simulink model "lane_keeping_fpga_in_the_loop"  (R2025b)
settings: Solver=ode1  StartTime=0.0  StopTime=30.0  RelTol=1e-3
model workspace (MAT data in the model file):
  firstWarning = 1
  originalScenarioChecksum = '9B63FD3C04BCEB1F00254244C35DE55B'
undefined symbols (not defined in the file): gray, Sim3dSensor
libraries: instrumentseriallib x3, simulink_extras x2, visiongeotforms x1, sim3dcameralib x1, sim3dlib x1, sim3dautolib x1
(part 2 of 2)

== matlab function lane_keeping_fpga_in_the_loop/LANE KEEPING PROCESS/lane_mask_corsia ==
  data: binary_img input; lane_mask output
function lane_mask = Keep_First_White_Point(binary_img)
%#codegen
% Input : binary_img [H x W] uint8
% Output: lane_mask [H x W] uint8
%
% Scopo:
%   Estrarre le due linee di corsia anche se entrambe si trovano
%   nella stessa metà dell'immagine.
%
% Convenzioni:
%   r = riga immagine, cresce verso il basso
%   c = colonna immagine, cresce verso destra
%   centro corsia = media delle due linee oppure linea singola +/- mezza corsia

[H,W] = size(binary_img);

lane_mask = zeros(H,W,'uint8');

% =========================================================
% Memoria centro dinamico tra frame
% =========================================================
persistent center_mem initialized

if isempty(initialized)
    center_mem = int32(W/2);
    initialized = true;
end

% =========================================================
% Parametri
% =========================================================
pixels_per_meter_x = 30.0;    % [px/m]
lane_width_m       = 3.5;     % [m]

lane_width_px = int32(round(lane_width_m * pixels_per_meter_x));
half_lane_px  = int32(round(0.5 * double(lane_width_px)));

% Accetto linee entro questa distanza dal centro stimato
% Più grande di una corsia perché la macchina può essere disallineata.
search_gate_px = int32(round(2.2 * double(lane_width_px)));

% Tolleranza sulla larghezza corsia
width_tol_px = 0.45 * double(lane_width_px);

% Salto massimo ammesso tra una riga e la successiva
max_shift = int32(round(0.18 * double(W)));

% Aggiornamento lento del centro per evitare oscillazioni
alpha_center = 0.10;

% Numero massimo di blob candidati per riga
MAX_CAND = 20;

% Memoria intra-frame
prev_left  = int32(0);
prev_right = int32(0);

has_left  = false;
has_right = false;

center = center_mem;

% =========================================================
% Scansione dal basso verso l'alto
% =========================================================
for r = H:-1:1

    % Saturazione centro
    if center < 1
        center = int32(1);
    end
    if center > W
        center = int32(W);
    end

    % =====================================================
    % 1) Trova tutti i blob bianchi sulla riga r
    % =====================================================
    cand = zeros(1,MAX_CAND,'int32');
    cand_count = int32(0);

    in_blob = false;
    blob_start = int32(0);

    for c = 1:W

        is_white = binary_img(r,c) > 0;

        if is_white && ~in_blob
            in_blob = true;
            blob_start = int32(c);
        end

        if (~is_white || c == W) && in_blob

            if is_white && c == W
                blob_end = int32(c);
            else
                blob_end = int32(c - 1);
            end

            blob_center = int32(round(0.5 * ...
                (double(blob_start) + double(blob_end))));

            if cand_count < MAX_CAND
                cand_count = cand_count + 1;
                cand(cand_count) = blob_center;
            end

            in_blob = false;
        end
    end

    % Se non ho candidati, mantengo centro precedente
    if cand_count == 0
        continue;
    end

    % =====================================================
    % 2) Selezione delle due linee migliori
    % =====================================================
    best_left  = int32(0);
    best_right = int32(0);
    found_pair = false;

    best_pair_cost = 1.0e12;

    % -----------------------------------------------------
    % Caso A: cerco una coppia con distanza circa lane_width_px
    % -----------------------------------------------------
    for i = 1:cand_count
        ci = cand(i);

        % Scarto candidati troppo lontani dal centro dinamico
        if abs(ci - center) > search_gate_px
            continue;
        end

        for j = 1:cand_count
            if j <= i
                continue;
            end

            cj = cand(j);

            if abs(cj - center) > search_gate_px
                continue;
            end

            % Ordino: left < right
            if ci < cj
                c_left  = ci;
                c_right = cj;
            else
                c_left  = cj;
                c_right = ci;
            end

            width_px = c_right - c_left;

            % Deve essere circa una larghezza corsia
            width_error = abs(double(width_px) - double(lane_width_px));

            if width_error > width_tol_px
                continue;
            end

            pair_center = int32(round(0.5 * ...
                (double(c_left) + double(c_right))));

            % Costo geometrico
            cost_width  = width_error;
            cost_center = abs(double(pair_center - center));

            % Costo di continuità se ho memoria
            cost_cont = 0.0;

            if has_left
                if abs(c_left - prev_left) > max_shift
                    cost_cont = cost_cont + 1.0e6;
                else
                    cost_cont = cost_cont + abs(double(c_left - prev_left));
                end
            end

            if has_right
                if abs(c_right - prev_right) > max_shift
                    cost_cont = cost_cont + 1.0e6;
                else
                    cost_cont = cost_cont + abs(double(c_right - prev_right));
                end
            end

            total_cost = 4.0*cost_width + 1.0*cost_center + 2.0*cost_cont;

            if total_cost < best_pair_cost
                best_pair_cost = total_cost;
                best_left  = c_left;
                best_right = c_right;
                found_pair = true;
            end
        end
    end

    % =====================================================
    % 3) Se non trovo coppia, scelgo la singola linea migliore
    % =====================================================
    found_single = false;
    best_single = int32(0);
    best_single_cost = 1.0e12;

    if ~found_pair

        for i = 1:cand_count
            ci = cand(i);

            if abs(ci - center) > search_gate_px
                continue;
            end

            % Costo base: vicinanza al centro dinamico
            cost = abs(double(ci - center));

            % Se ho una linea precedente, privilegio la continuità
            if has_left && has_right
                dL = abs(ci - prev_left);
                dR = abs(ci - prev_right);
                cost = cost + 2.0 * double(min(dL,dR));
            elseif has_left
                cost = cost + 2.0 * double(abs(ci - prev_left));
            elseif has_right
                cost = cost + 2.0 * double(abs(ci - prev_right));
            end

            if cost < best_single_cost
                best_single_cost = cost;
                best_single = ci;
                found_single = true;
            end
        end
    end

    % =====================================================
    % 4) Scrittura output e aggiornamento centro
    % =====================================================
    center_new = center;

    if found_pair

        % Disegno entrambe le linee
        lane_mask(r,best_left)  = uint8(255);
        lane_mask(r,best_right) = uint8(255);

        prev_left  = best_left;
        prev_right = best_right;

        has_left  = true;
        has_right = true;

        center_new = int32(round(0.5 * ...
            (double(best_left) + double(best_right))));

    elseif found_single

        % Disegno la singola linea trovata
        lane_mask(r,best_single) = uint8(255);

        % Devo decidere se è linea sinistra o destra della corsia.
        % Ipotesi:
        %   se la linea è a sinistra del centro stimato, allora è left;
        %   se è a destra, allora è right.
        %
        % Nota: anche se entrambe le linee stanno nella stessa metà immagine,
        % questa scelta resta coerente rispetto al centro dinamico stimato.

        if best_single < center

            % Linea sinistra vista
            prev_left = best_single;
            has_left = true;

            center_new = best_single + half_lane_px;

        else

            % Linea destra vista
            prev_right = best_single;
            has_right = true;

            center_new = best_single - half_lane_px;

        end

    else

        center_new = center;

    end

    % =====================================================
    % 5) Filtro del centro dinamico
    % =====================================================
    center = int32(round((1.0 - alpha_center)*double(center) + ...
                         alpha_center*double(center_new)));

    if center < 1
        center = int32(1);
    end
    if center > W
        center = int32(W);
    end

end

% =========================================================
% Salvo memoria per frame successivo
% =========================================================
center_mem = center;

end

== matlab function lane_keeping_fpga_in_the_loop/LANE KEEPING PROCESS/rotazione corsia/fitting_lnes ==
  data: lane_img output; lane_mask input; validL output; aL output; bL output; cL output; validR output; aR output; bR output; cR output
function [lane_img, validL, aL, bL, cL, validR, aR, bR, cR] = Fit_Left_Right_Lanes(lane_mask)
%#codegen

[H,W] = size(lane_mask);
lane_img = lane_mask;

center_fixed = double(W)/2.0;

validL = false;
validR = false;

aL = 0.0;
bL = 0.0;
cL = 0.0;

aR = 0.0;
bR = 0.0;
cR = 0.0;

[validL1, validR1, aL1, bL1, cL1, aR1, bR1, cR1] = ...
    fit_lanes_internal(lane_mask, false, ...
                       0.0, 0.0, 0.0, ...
                       0.0, 0.0, 0.0, ...
                       center_fixed);

if ~(validL1 && validR1)

    validL = validL1;
    validR = validR1;

    aL = aL1;
    bL = bL1;
    cL = cL1;

    aR = aR1;
    bR = bR1;
    cR = cR1;

    return;
end

[validL2, validR2, aL2, bL2, cL2, aR2, bR2, cR2] = ...
    fit_lanes_internal(lane_mask, true, ...
                       aL1, bL1, cL1, ...
                       aR1, bR1, cR1, ...
                       center_fixed);

if validL2 && validR2

    validL = validL2;
    validR = validR2;

    aL = aL2;
    bL = bL2;
    cL = cL2;

    aR = aR2;
    bR = bR2;
    cR = cR2;

else

    validL = validL1;
    validR = validR1;

    aL = aL1;
    bL = bL1;
    cL = cL1;

    aR = aR1;
    bR = bR1;
    cR = cR1;

end

end


function [validL, validR, aL, bL, cL, aR, bR, cR] = ...
    fit_lanes_internal(lane_mask, use_corrected_center, ...
                       aLprev, bLprev, cLprev, ...
                       aRprev, bRprev, cRprev, ...
                       center_fixed)
%#codegen

persistent center_mem initialized

[H,W] = size(lane_mask);

if isempty(initialized)
    center_mem = center_fixed;
    initialized = true;
end

validL = false;
validR = false;

aL = 0.0;
bL = 0.0;
cL = 0.0;

aR = 0.0;
bR = 0.0;
cR = 0.0;

% =========================================================
% Parametri fisici
% =========================================================
pixels_per_meter_x = 30.0;
lane_width_m       = 3.5;

lane_width_px      = lane_width_m * pixels_per_meter_x;
half_lane_width_px = 0.5 * lane_width_px;

% Tolleranza per capire se distanza = 1 corsia o 2 corsie
width_tol_px = 0.35 * lane_width_px;

% Gate: accetto punti entro 1 corsia dal centro stimato
center_gate_px = lane_width_px;

% Media mobile centro
alpha_center = 0.20;

% =========================================================
% Accumulatori sinistra
% =========================================================
nL = 0.0;
SyL = 0.0;
Sy2L = 0.0;
Sy3L = 0.0;
Sy4L = 0.0;
SxL = 0.0;
SxyL = 0.0;
Sxy2L = 0.0;

% =========================================================
% Accumulatori destra
% =========================================================
nR = 0.0;
SyR = 0.0;
Sy2R = 0.0;
Sy3R = 0.0;
Sy4R = 0.0;
SxR = 0.0;
SxyR = 0.0;
Sxy2R = 0.0;

for r = 1:H

    y = double(r);

    if use_corrected_center

        xLprev = aLprev*y*y + bLprev*y + cLprev;
        xRprev = aRprev*y*y + bRprev*y + cRprev;

        measured_width = xRprev - xLprev;

        is_one_lane = abs(measured_width - lane_width_px) <= width_tol_px;
        is_two_lane = abs(measured_width - 2.0*lane_width_px) <= width_tol_px;

        if is_one_lane

            % Caso corretto: due linee della stessa corsia
            center_fit = 0.5*(xLprev + xRprev);

        elseif is_two_lane

            % Caso esterno: le due linee sono separate da circa 2 corsie
            dist_to_left  = abs(center_mem - xLprev);
            dist_to_right = abs(center_mem - xRprev);

            if dist_to_right < dist_to_left
                % linea più vicina è la destra:
                % centro corsia = mezzo lane width a sinistra della destra
                center_fit = xRprev - half_lane_width_px;
            else
                % linea più vicina è la sinistra:
                % centro corsia = mezzo lane width a destra della sinistra
                center_fit = xLprev + half_lane_width_px;
            end

        else

            % Caso incerto: mantengo memoria
            center_fit = center_mem;

        end

        % Media mobile
        center_mem = (1.0 - alpha_center)*center_mem + alpha_center*center_fit;

        center_dyn = center_mem;

        if center_dyn < 1.0
            center_dyn = 1.0;
        end

        if center_dyn > double(W)
            center_dyn = double(W);
        end

    else

        center_dyn = center_fixed;

    end

    for col = 1:W

        if lane_mask(r,col) > 0

            x = double(col);

            y2 = y*y;
            y3 = y2*y;
            y4 = y2*y2;

            assign_left = false;
            assign_right = false;

            if ~use_corrected_center

                if x < center_dyn
                    assign_left = true;
                else
                    assign_right = true;
                end

            else

                dist_from_center = abs(x - center_dyn);

                if dist_from_center <= center_gate_px

                    if x < center_dyn
                        assign_left = true;
                    else
                        assign_right = true;
                    end

                end
            end

            if assign_left

                nL = nL + 1.0;

                SyL   = SyL   + y;
                Sy2L  = Sy2L  + y2;
                Sy3L  = Sy3L  + y3;
                Sy4L  = Sy4L  + y4;

                SxL   = SxL   + x;
                SxyL  = SxyL  + x*y;
                Sxy2L = Sxy2L + x*y2;

            elseif assign_right

                nR = nR + 1.0;

                SyR   = SyR   + y;
                Sy2R  = Sy2R  + y2;
                Sy3R  = Sy3R  + y3;
                Sy4R  = SyR + y4;   % CORRETTO SOTTO
                Sy4R  = Sy4R - SyR + y4;

                SxR   = SxR   + x;
                SxyR  = SxyR  + x*y;
                Sxy2R = Sxy2R + x*y2;

            end
        end
    end
end

if nL >= 6.0

    [okL, aaL, bbL, ccL] = solve_parabola_ls( ...
        SyL, Sy2L, Sy3L, Sy4L, ...
        SxL, SxyL, Sxy2L, nL);

    if okL
        aL = aaL;
        bL = bbL;
        cL = ccL;
        validL = true;
    end
end

if nR >= 6.0

    [okR, aaR, bbR, ccR] = solve_parabola_ls( ...
        SyR, Sy2R, Sy3R, Sy4R, ...
        SxR, SxyR, Sxy2R, nR);

    if okR
        aR = aaR;
        bR = bbR;
        cR = ccR;
        validR = true;
    end
end

end


function [ok, a, b, c] = solve_parabola_ls( ...
    Sy, Sy2, Sy3, Sy4, Sx, Sxy, Sxy2, n)
%#codegen

ok = false;

a = 0.0;
b = 0.0;
c = 0.0;

A11 = Sy4;
A12 = Sy3;
A13 = Sy2;

A21 = Sy3;
A22 = Sy2;
A23 = Sy;

A31 = Sy2;
A32 = Sy;
A33 = n;

B1 = Sxy2;
B2 = Sxy;
B3 = Sx;

detA = A11*(A22*A33 - A23*A32) ...
     - A12*(A21*A33 - A23*A31) ...
     + A13*(A21*A32 - A22*A31);

if abs(detA) > 1e-9

    detA1 = B1*(A22*A33 - A23*A32) ...
          - A12*(B2*A33 - A23*B3) ...
          + A13*(B2*A32 - A22*B3);

    detA2 = A11*(B2*A33 - A23*B3) ...
          - B1*(A21*A33 - A23*A31) ...
          + A13*(A21*B3 - B2*A31);

    detA3 = A11*(A22*B3 - B2*A32) ...
          - A12*(A21*B3 - B2*A31) ...
          + B1*(A21*A32 - A22*A31);

    a = detA1 / detA;
    b = detA2 / detA;
    c = detA3 / detA;

    ok = true;
end

end
